simulink model "helicopter_LINEARIZED"  (R2017b)
settings: Solver=FixedStepAuto  StartTime=0.0  StopTime=10  FixedStep=0.0001  RelTol=1e-3
values from neighbouring files (symbols this model uses):
  epsilon_m = 0.01    [helicopter_params_LINEARIZED.m]
  Euler0 = [0.0,0.2,0.2]'    [helicopter_params_LINEARIZED.m]
  g = 9.81    [helicopter_params_LINEARIZED.m]
  J1 = 10^(-3)    (= 0.001)    [helicopter_params_LINEARIZED.m]
  J2 = 10^(-3)    (= 0.001)    [helicopter_params_LINEARIZED.m]
  J3 = 10^(-3)    (= 0.001)    [helicopter_params_LINEARIZED.m]
  K1 = [-0.0024   -0.0191    0.0543    0.0141]    [helicopter_params_LINEARIZED.m]
  K2 = [0.0024    0.0191    0.0543    0.0141]    [helicopter_params_LINEARIZED.m]
  K3 = [-0.0236   -1.3500]    [helicopter_params_LINEARIZED.m]
  K4 = [0.0200    0.3000] *20    [helicopter_params_LINEARIZED.m]
  l = 0.001    [helicopter_params_LINEARIZED.m]
  m = 4.5    [helicopter_params_LINEARIZED.m]
  p0 = [0.1,0.2,0.3]'    [helicopter_params_LINEARIZED.m]
  Q = ke5 * sqrt(m*g)    [helicopter_params_LINEARIZED.m]
  v0 = [0.0,0.0,0.0]'    [helicopter_params_LINEARIZED.m]
  w0 = [0.0,0.0,0.0]'    [helicopter_params_LINEARIZED.m]
settings Model: Creator=Marco  LastModifiedBy=Marco

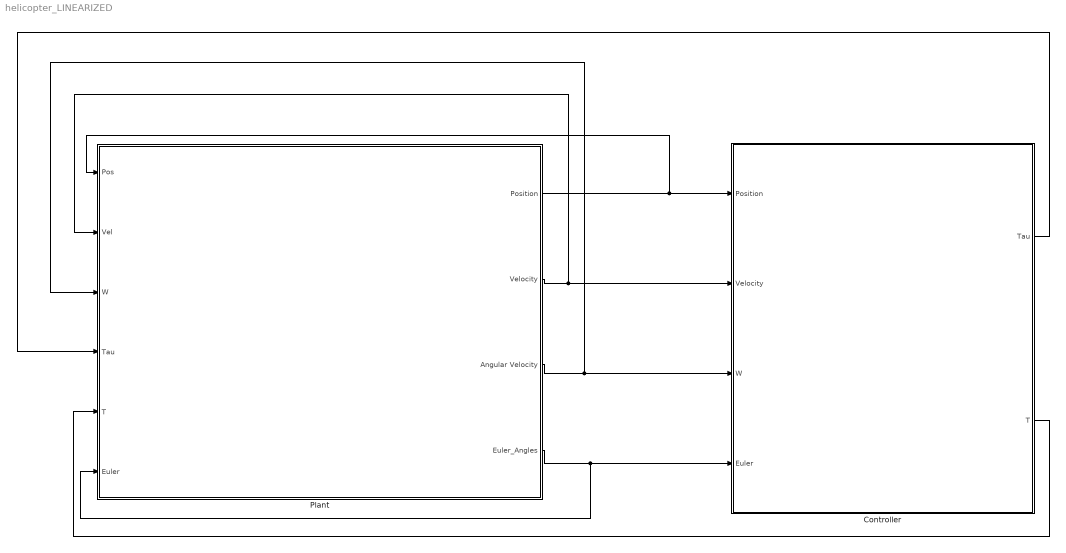
== system helicopter_LINEARIZED ==
  Controller : Subsystem
  Plant : Subsystem
  wires:
  Plant/1(Position) -> Plant/1(Pos), Controller/1(Position)
  Plant/2(Velocity) -> Plant/2(Vel), Controller/2(Velocity)
  Plant/3(Angular Velocity) -> Plant/3(W), Controller/3(W)
  Plant/4(Euler_Angles) -> Plant/6(Euler), Controller/4(Euler)
  Controller/2(T) -> Plant/5(T)
  Controller/1(Tau) -> Plant/4(Tau)

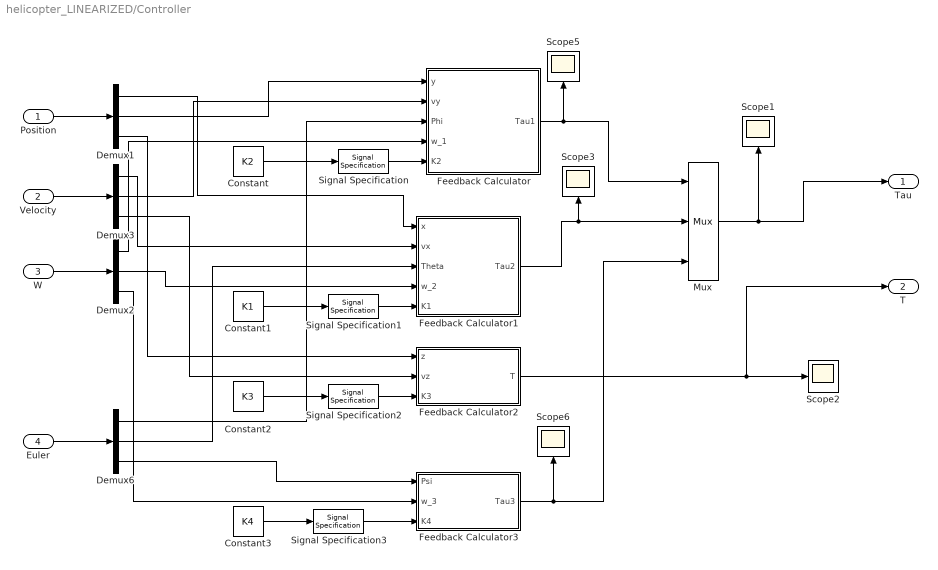
== system helicopter_LINEARIZED/Controller ==
  Position : Inport
  Velocity : Inport  Port=2
  W : Inport  Port=3
  Euler : Inport  Port=4
  Constant : Constant  Value=K2
  Constant1 : Constant  Value=K1
  Constant2 : Constant  Value=K3
  Constant3 : Constant  Value=K4
  Demux{1..3,6} (4 alike) : Demux  Outputs=3
  Feedback Calculator : MATLAB Function  TreatAsAtomicUnit=on
  Feedback Calculator1 : MATLAB Function  TreatAsAtomicUnit=on
  Feedback Calculator2 : MATLAB Function  TreatAsAtomicUnit=on
  Feedback Calculator3 : MATLAB Function  TreatAsAtomicUnit=on
  Mux : Mux  Inputs=3
  Scope{1..3,5..6} (5 alike) : Scope
  Signal Specification : SignalSpecification  Dimensions=[1,4]
  Signal Specification1 : SignalSpecification  Dimensions=[1,4]
  Signal Specification2 : SignalSpecification  Dimensions=[1,2]
  Signal Specification3 : SignalSpecification  Dimensions=[1,2]
  Tau : Outport
  T : Outport  Port=2
  wires:
  Feedback Calculator/1(Tau1) -> Scope5/1, Mux/1
  Feedback Calculator1/1(Tau2) -> Scope3/1, Mux/2
  Feedback Calculator3/1(Tau3) -> Scope6/1, Mux/3
  Feedback Calculator2/1(T) -> Scope2/1, T/1
  Mux/1 -> Scope1/1, Tau/1
  W/1 -> Demux2/1
  Position/1 -> Demux1/1
  Velocity/1 -> Demux3/1
  Euler/1 -> Demux6/1
  Demux1/2 -> Feedback Calculator/1(y)
  Demux3/2 -> Feedback Calculator/2(vy)
  Demux6/1 -> Feedback Calculator/3(Phi)
  Demux1/1 -> Feedback Calculator1/1(x)
  Demux3/1 -> Feedback Calculator1/2(vx)
  Demux6/2 -> Feedback Calculator1/3(Theta)
  Demux2/2 -> Feedback Calculator1/4(w_2)
  Demux2/1 -> Feedback Calculator/4(w_1)
  Demux3/3 -> Feedback Calculator2/2(vz)
  Demux2/3 -> Feedback Calculator3/2(w_3)
  Constant/1 -> Signal Specification/1
  Constant1/1 -> Signal Specification1/1
  Constant2/1 -> Signal Specification2/1
  Constant3/1 -> Signal Specification3/1
  Demux6/3 -> Feedback Calculator3/1(Psi)
  Demux1/3 -> Feedback Calculator2/1(z)
  Signal Specification/1 -> Feedback Calculator/5(K2)
  Signal Specification1/1 -> Feedback Calculator1/5(K1)
  Signal Specification2/1 -> Feedback Calculator2/3(K3)
  Signal Specification3/1 -> Feedback Calculator3/3(K4)

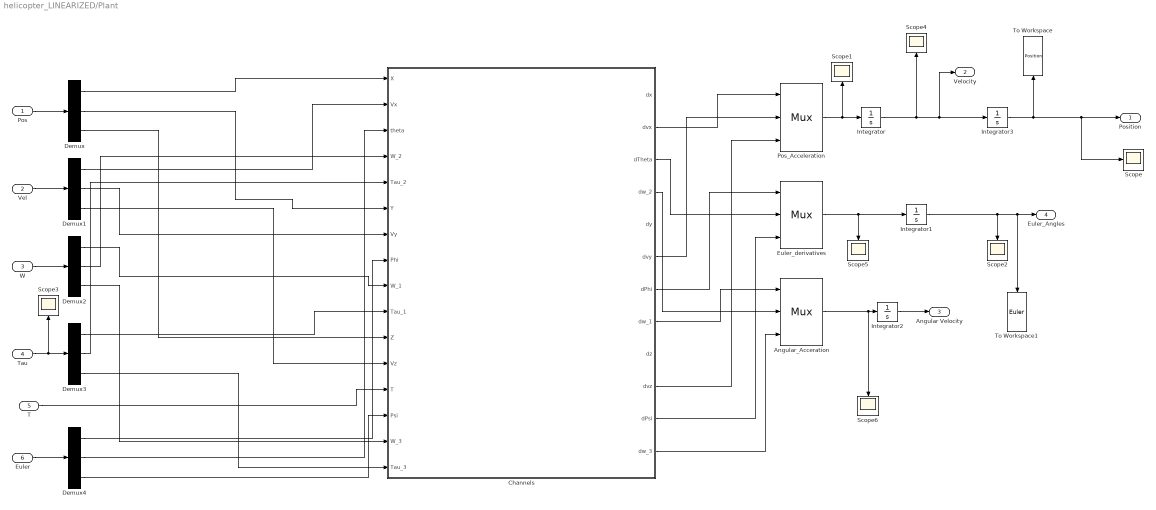
== system helicopter_LINEARIZED/Plant ==
  Pos : Inport
  Vel : Inport  Port=2
  W : Inport  Port=3
  Tau : Inport  Port=4
  T : Inport  Port=5
  Euler : Inport  Port=6
  Angular_Acceration : Mux  Inputs=3
  Channels : Subsystem
  Demux{,1..4} (5 alike) : Demux  Outputs=3
  Euler_derivatives : Mux  Inputs=3
  Integrator : Integrator  InitialCondition=v0
  Integrator1 : Integrator  InitialCondition=Euler0
  Integrator2 : Integrator  InitialCondition=w0
  Integrator3 : Integrator  InitialCondition=p0
  Pos_Acceleration : Mux  Inputs=3
  Scope{,1..6} (7 alike) : Scope
  To Workspace : ToWorkspace  VariableName=Position  SampleTime=-1
  To Workspace1 : ToWorkspace  VariableName=Euler  SampleTime=-1
  Position : Outport
  Velocity : Outport  Port=2
  Angular Velocity : Outport  Port=3
  Euler_Angles : Outport  Port=4
  wires:
  Pos/1 -> Demux/1
  Vel/1 -> Demux1/1
  W/1 -> Demux2/1
  Tau/1 -> Scope3/1, Demux3/1
  Euler/1 -> Demux4/1
  T/1 -> Channels/13(T)
  Demux/1 -> Channels/1(X)
  Demux/2 -> Channels/6(Y)
  Demux/3 -> Channels/11(Z)
  Demux1/1 -> Channels/2(Vx)
  Demux1/2 -> Channels/7(Vy)
  Demux1/3 -> Channels/12(Vz)
  Demux2/1 -> Channels/9(W_1)
  Demux2/2 -> Channels/4(W_2)
  Demux2/3 -> Channels/15(W_3)
  Demux3/1 -> Channels/10(Tau_1)
  Demux3/2 -> Channels/5(Tau_2)
  Demux3/3 -> Channels/16(Tau_3)
  Demux4/1 -> Channels/8(Phi)
  Demux4/2 -> Channels/3(theta)
  Demux4/3 -> Channels/14(Psi)
  Channels/2(dvx) -> Pos_Acceleration/1
  Channels/6(dvy) -> Pos_Acceleration/2
  Channels/10(dvz) -> Pos_Acceleration/3
  Channels/7(dPhi) -> Euler_derivatives/1
  Channels/3(dTheta) -> Euler_derivatives/2
  Channels/11(dPsi) -> Euler_derivatives/3
  Channels/8(dw_1) -> Angular_Acceration/1
  Channels/4(dw_2) -> Angular_Acceration/2
  Channels/12(dw_3) -> Angular_Acceration/3
  Pos_Acceleration/1 -> Integrator/1, Scope1/1
  Euler_derivatives/1 -> Scope5/1, Integrator1/1
  Integrator/1 -> Velocity/1, Integrator3/1, Scope4/1
  Integrator1/1 -> Scope2/1, To Workspace1/1, Euler_Angles/1
  Angular_Acceration/1 -> Scope6/1, Integrator2/1
  Integrator2/1 -> Angular Velocity/1
  Integrator3/1 -> To Workspace/1, Scope/1, Position/1

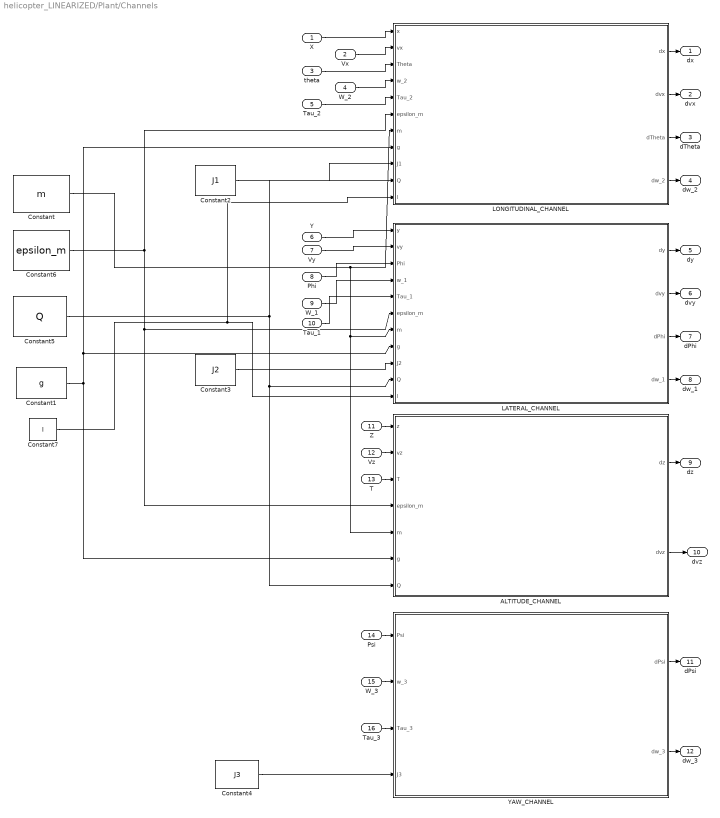
== system helicopter_LINEARIZED/Plant/Channels ==
  X : Inport
  Vx : Inport  Port=2
  theta : Inport  Port=3
  W_2 : Inport  Port=4
  Tau_2 : Inport  Port=5
  Y : Inport  Port=6
  Vy : Inport  Port=7
  Phi : Inport  Port=8
  W_1 : Inport  Port=9
  Tau_1 : Inport  Port=10
  Z : Inport  Port=11
  Vz : Inport  Port=12
  T : Inport  Port=13
  Psi : Inport  Port=14
  W_3 : Inport  Port=15
  Tau_3 : Inport  Port=16
  ALTITUDE_CHANNEL : MATLAB Function  TreatAsAtomicUnit=on
  Constant : Constant  Value=m
  Constant1 : Constant  Value=g
  Constant2 : Constant  Value=J1
  Constant3 : Constant  Value=J2
  Constant4 : Constant  Value=J3
  Constant5 : Constant  Value=Q
  Constant6 : Constant  Value=epsilon_m
  Constant7 : Constant  Value=l
  LATERAL_CHANNEL : MATLAB Function  TreatAsAtomicUnit=on
  LONGITUDINAL_CHANNEL : MATLAB Function  TreatAsAtomicUnit=on
  YAW_CHANNEL : MATLAB Function  TreatAsAtomicUnit=on
  dx : Outport
  dvx : Outport  Port=2
  dTheta : Outport  Port=3
  dw_2 : Outport  Port=4
  dy : Outport  Port=5
  dvy : Outport  Port=6
  dPhi : Outport  Port=7
  dw_1 : Outport  Port=8
  dz : Outport  Port=9
  dvz : Outport  Port=10
  dPsi : Outport  Port=11
  dw_3 : Outport  Port=12
  wires:
  LATERAL_CHANNEL/1(dy) -> dy/1
  LATERAL_CHANNEL/2(dvy) -> dvy/1
  LATERAL_CHANNEL/4(dw_1) -> dw_1/1
  Tau_2/1 -> LONGITUDINAL_CHANNEL/5(Tau_2)
  Constant2/1 -> LONGITUDINAL_CHANNEL/9(J1)
  Z/1 -> ALTITUDE_CHANNEL/1(z)
  LONGITUDINAL_CHANNEL/4(dw_2) -> dw_2/1
  Constant4/1 -> YAW_CHANNEL/4(J3)
  Psi/1 -> YAW_CHANNEL/1(Psi)
  Constant1/1 -> LONGITUDINAL_CHANNEL/8(g), LATERAL_CHANNEL/8(g), ALTITUDE_CHANNEL/6(g)
  LATERAL_CHANNEL/3(dPhi) -> dPhi/1
  Vz/1 -> ALTITUDE_CHANNEL/2(vz)
  YAW_CHANNEL/1(dPsi) -> dPsi/1
  LONGITUDINAL_CHANNEL/3(dTheta) -> dTheta/1
  Phi/1 -> LATERAL_CHANNEL/3(Phi)
  Tau_1/1 -> LATERAL_CHANNEL/5(Tau_1)
  Tau_3/1 -> YAW_CHANNEL/3(Tau_3)
  YAW_CHANNEL/2(dw_3) -> dw_3/1
  Y/1 -> LATERAL_CHANNEL/1(y)
  W_1/1 -> LATERAL_CHANNEL/4(w_1)
  X/1 -> LONGITUDINAL_CHANNEL/1(x)
  Constant/1 -> ALTITUDE_CHANNEL/5(m), LATERAL_CHANNEL/7(m), LONGITUDINAL_CHANNEL/7(m)
  T/1 -> ALTITUDE_CHANNEL/3(T)
  W_3/1 -> YAW_CHANNEL/2(w_3)
  Constant6/1 -> LONGITUDINAL_CHANNEL/6(epsilon_m), ALTITUDE_CHANNEL/4(epsilon_m), LATERAL_CHANNEL/6(epsilon_m)
  Constant5/1 -> LONGITUDINAL_CHANNEL/10(Q), LATERAL_CHANNEL/10(Q), ALTITUDE_CHANNEL/7(Q)
  ALTITUDE_CHANNEL/1(dz) -> dz/1
  W_2/1 -> LONGITUDINAL_CHANNEL/4(w_2)
  Vy/1 -> LATERAL_CHANNEL/2(vy)
  theta/1 -> LONGITUDINAL_CHANNEL/3(Theta)
  Vx/1 -> LONGITUDINAL_CHANNEL/2(vx)
  LONGITUDINAL_CHANNEL/2(dvx) -> dvx/1
  LONGITUDINAL_CHANNEL/1(dx) -> dx/1
  Constant3/1 -> LATERAL_CHANNEL/9(J2)
  Constant7/1 -> LATERAL_CHANNEL/11(l), LONGITUDINAL_CHANNEL/11(l)
  ALTITUDE_CHANNEL/2(dvz) -> dvz/1

== matlab function helicopter_LINEARIZED/Plant/Channels/LATERAL_CHANNEL ==
  data: y input; vy input; Phi input; w_1 input; Tau_1 input; dy output; dvy output; dPhi output; dw_1 output; epsilon_m input; m input; g input; J2 input; Q input; l input
function [dy,dvy,dPhi,dw_1] = SISO2(y,vy,Phi,w_1,Tau_1,epsilon_m,m,g,J2,Q,l)
dy = vy;
dvy = -(Q/m) * vy + g * Phi - (1/(m*l)) * Tau_1;
dPhi = w_1;
dw_1 = epsilon_m * Q * (1/J2) * vy + (1/J2) * Tau_1;

== matlab function helicopter_LINEARIZED/Plant/Channels/LONGITUDINAL_CHANNEL ==
  data: x input; vx input; Theta input; w_2 input; Tau_2 input; dx output; dvx output; dTheta output; dw_2 output; epsilon_m input; m input; g input; J1 input; Q input; l input
function [dx,dvx,dTheta,dw_2] = SISO1(x,vx,Theta,w_2,Tau_2,epsilon_m,m,g,J1,Q,l)
dx = vx;
dvx = -(Q/m) * vx - g * Theta + (1/(m*l)) * Tau_2;
dTheta = w_2;
dw_2 = -epsilon_m * Q * (1/J1) * vx + (1/J1) * Tau_2;

== matlab function helicopter_LINEARIZED/Plant/Channels/ALTITUDE_CHANNEL ==
  data: z input; vz input; T input; dz output; dvz output; epsilon_m input; m input; g input; Q input
function [dz,dvz] = SISO3(z,vz,T,epsilon_m,m,g,Q)
dz = vz;
%dvz = -(Q/m) * z + (1/m) * (T - m*g)
dvz = -(Q/m) * z + (1/m) * (T);

== matlab function helicopter_LINEARIZED/Plant/Channels/YAW_CHANNEL ==
  data: Psi input; w_3 input; dPsi output; dw_3 output; Tau_3 input; J3 input
function [dPsi,dw_3] = SISO4(Psi,w_3,Tau_3,J3)
dPsi = w_3;
dw_3 = (1/J3) * Tau_3;

== matlab function helicopter_LINEARIZED/Controller/Feedback Calculator ==
  data: y input; Tau1 output; vy input; Phi input; w_1 input; K2 input
function Tau1 = Tau1(y,vy,Phi,w_1,K2)
Tau1 = zeros(1,1);
state = zeros(4,1);
state = [y;vy;Phi;w_1];
Tau1 = -K2 * state;

== matlab function helicopter_LINEARIZED/Controller/Feedback Calculator1 ==
  data: x input; Tau2 output; vx input; Theta input; w_2 input; K1 input
function Tau2 = Tau2(x,vx,Theta,w_2,K1)
Tau2 = zeros(1,1);
state = zeros(4,1);
state = [x;vx;Theta;w_2];
Tau2 = -K1 * state;

== matlab function helicopter_LINEARIZED/Controller/Feedback Calculator2 ==
  data: z input; T output; vz input; K3 input
function T = Thrust(z,vz,K3)
T = zeros(1,1);
state = zeros(2,1);
state = [z;vz];
T = K3 * state;

== matlab function helicopter_LINEARIZED/Controller/Feedback Calculator3 ==
  data: Psi input; Tau3 output; w_3 input; K4 input
function Tau3 = Tau3(Psi,w_3,K4)
Tau3 = zeros(1,1);
state = zeros(2,1);
state = [Psi;w_3];
Tau3 = -K4 * state;
